simulink model "L3P1A4b"  (R2023a)
settings: Solver=VariableStepAuto  StartTime=0.0  StopTime=100  RelTol=1e-3
settings Model: Creator=rqouta  LastModifiedBy=rqouta

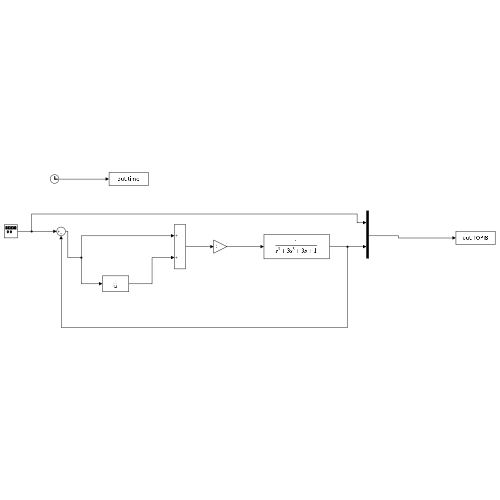
[thumbnail: Simulink's stored preview of the top-level diagram]
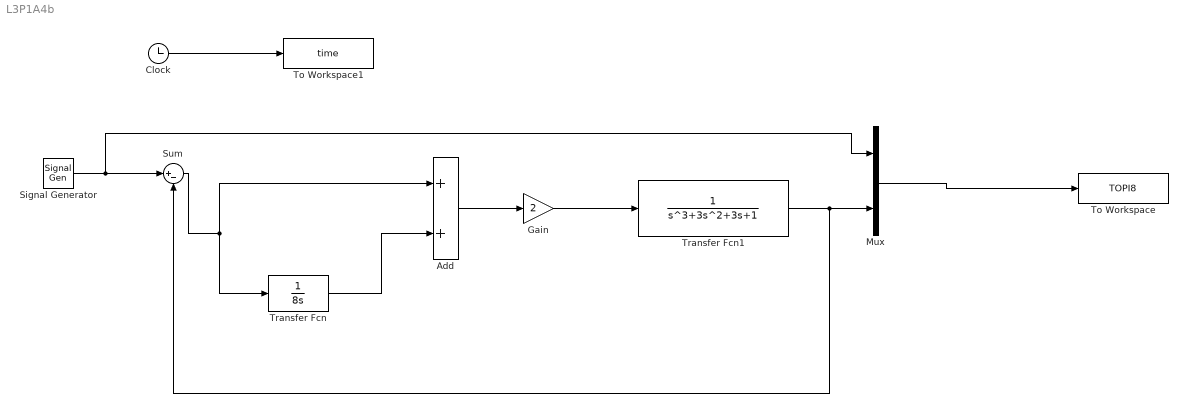
== system L3P1A4b ==
  Add : Sum
  Clock : Clock
  Gain : Gain  Gain=2
  Mux : Mux  Inputs=2
  Signal Generator : SignalGenerator  WaveForm=square  Frequency=0.01
  Sum : Sum  Inputs=|+-
  To Workspace : ToWorkspace  VariableName=TOPI8  SampleTime=-1
  To Workspace1 : ToWorkspace  VariableName=time  SampleTime=-1
  Transfer Fcn : TransferFcn  Denominator=[8 0]
  Transfer Fcn1 : TransferFcn  Denominator=[1 3 3 1]
  wires:
  Gain/1 -> Transfer Fcn1/1
  Clock/1 -> To Workspace1/1
  Add/1 -> Gain/1
  Signal Generator/1 -> Mux/1, Sum/1
  Mux/1 -> To Workspace/1
  Transfer Fcn/1 -> Add/2
  Transfer Fcn1/1 -> Sum/2, Mux/2
  Sum/1 -> Transfer Fcn/1, Add/1
